simulink model "lab3_ekf_simulation"  (R2023b)
settings: Solver=FixedStepAuto  StartTime=0.0  StopTime=30  RelTol=1e-3
values from neighbouring files (symbols this model uses):
  A_model = A    [lab3_ekf_formulation.m]    (also in lab3_ekf_formulation_vel.m)
  F_linear = A    [lab3_ekf_formulation.m]    (also in lab3_ekf_formulation_vel.m)
  P_init = Q    [lab3_ekf_formulation.m]    (also in lab3_ekf_formulation_vel.m)
  Q = [1 alpha 1/2*alpha ; alpha alpha^2 1/2*alpha^2 ;      1/2*alpha 1/2*alpha^2 1/4*alpha^4]*expected_x_std^2*1e-3    [lab3_ekf_formulation.m]    (also in lab3_ekf_formulation_no_simulink.m = diag([0.2 0.4 1.0])*expected_x_std^2; lab3_ekf_formulation_vel.m = diag([0.2 0.4]))
  R = sensor_noise_var    [lab3_ekf_formulation.m]    (also in lab3_ekf_formulation_no_simulink.m; lab3_ekf_formulation_vel.m)
  sensor_coeffs = coeffs    [lab3_ekf_formulation.m]    (also in lab3_ekf_formulation_no_simulink.m; lab3_ekf_formulation_vel.m)
  T_ekf = 1/nyquist_freq    (= 0.153846153846)    [lab3_ekf_formulation.m]    (also in lab3_ekf_formulation_no_simulink.m = 0.133333333333; lab3_ekf_formulation_vel.m = 1E-4*floor(1/nyquist_freq*1E4))
  x_init = zeros(3,1)    [lab3_ekf_formulation.m]    (also in lab3_ekf_formulation_vel.m = zeros(2,1))
libraries: simulink x2
settings Model: Creator=samuel  LastModifiedBy=samuel

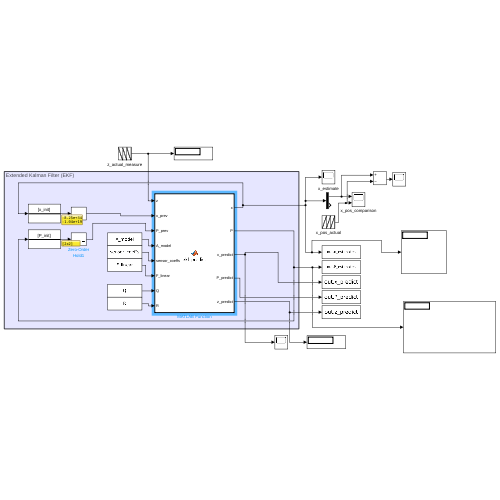
[thumbnail: Simulink's stored preview of the top-level diagram]
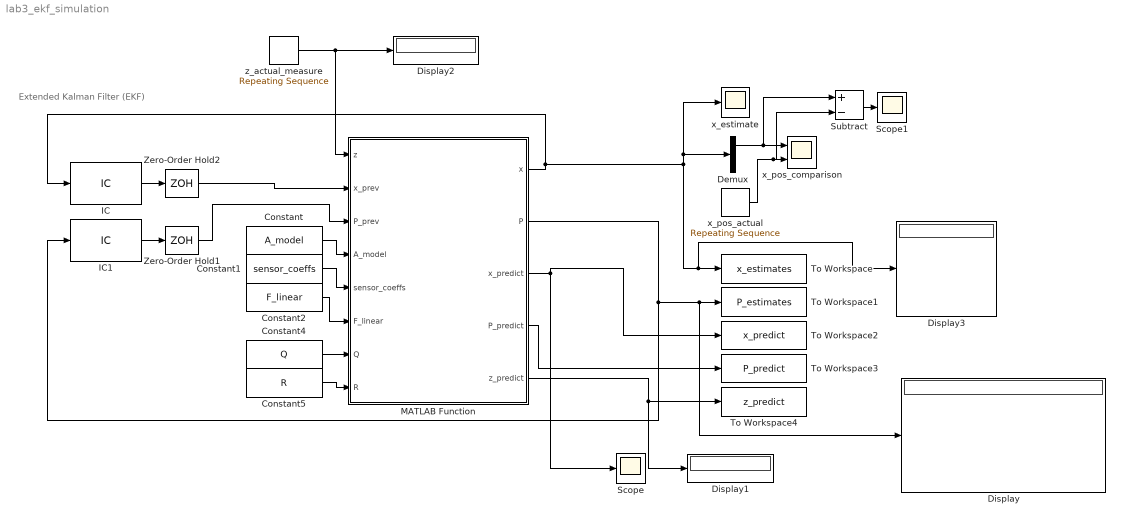
== system lab3_ekf_simulation ==
  note: Extended Kalman Filter (EKF)
  Constant : Constant  Value=A_model  VectorParams1D=off
  Constant1 : Constant  Value=sensor_coeffs
  Constant2 : Constant  Value=F_linear  VectorParams1D=off
  Constant4 : Constant  Value=Q  VectorParams1D=off
  Constant5 : Constant  Value=R  VectorParams1D=off
  Demux : Demux  Outputs=2
  Display{,1..3} (4 alike) : Display
  IC : InitialCondition  Value=x_init
  IC1 : InitialCondition  Value=P_init
  MATLAB Function : MATLAB Function  TreatAsAtomicUnit=on
  Scope : Scope
  Scope1 : Scope
  Subtract : Sum  Inputs=+-
  To Workspace : ToWorkspace  VariableName=x_estimates  SampleTime=-1
  To Workspace1 : ToWorkspace  VariableName=P_estimates  SampleTime=-1
  To Workspace2 : ToWorkspace  VariableName=x_predict  SampleTime=-1
  To Workspace3 : ToWorkspace  VariableName=P_predict  SampleTime=-1
  To Workspace4 : ToWorkspace  VariableName=z_predict  SampleTime=-1
  Zero-Order Hold1 : ZeroOrderHold  SampleTime=T_ekf
  Zero-Order Hold2 : ZeroOrderHold  SampleTime=T_ekf
  x_estimate : Scope
  x_pos_actual : simulink/Sources/Repeating Sequence  rep_seq_t=t_actual  rep_seq_y=x_pos_actual
  x_pos_comparison : Scope  NumInputPorts=2
  z_actual_measure : simulink/Sources/Repeating Sequence  rep_seq_t=t_actual  rep_seq_y=z_actual_measure
  wires:
  MATLAB Function/2(P) -> Display/1, To Workspace1/1, IC1/1
  MATLAB Function/1(x) -> x_estimate/1, Demux/1, Display3/1, To Workspace/1, IC/1
  z_actual_measure/1 -> MATLAB Function/1(z), Display2/1
  Demux/1 -> Subtract/1, x_pos_comparison/1
  x_pos_actual/1 -> Subtract/2, x_pos_comparison/2
  Constant/1 -> MATLAB Function/4(A_model)
  Constant5/1 -> MATLAB Function/8(R)
  Constant4/1 -> MATLAB Function/7(Q)
  Constant2/1 -> MATLAB Function/6(F_linear)
  Constant1/1 -> MATLAB Function/5(sensor_coeffs)
  IC/1 -> Zero-Order Hold2/1
  IC1/1 -> Zero-Order Hold1/1
  Zero-Order Hold1/1 -> MATLAB Function/3(P_prev)
  Zero-Order Hold2/1 -> MATLAB Function/2(x_prev)
  MATLAB Function/3(x_predict) -> To Workspace2/1, Scope/1
  MATLAB Function/4(P_predict) -> To Workspace3/1
  MATLAB Function/5(z_predict) -> Display1/1, To Workspace4/1
  Subtract/1 -> Scope1/1

== matlab function lab3_ekf_simulation/MATLAB Function ==
  data: z input; x_prev input; P_prev input; x output; P output; A_model input; sensor_coeffs input; F_linear input; Q input; R input; x_predict output; P_predict output; z_predict output
function [x,P,x_predict,P_predict,z_predict] = ekf_predict(z,x_prev,P_prev,...
    A_model,sensor_coeffs,F_linear,Q,R)

x = zeros(size(x_prev));
P = zeros(size(P_prev));

% sensor coefficients
a = sensor_coeffs(1);
b = sensor_coeffs(2);
c = sensor_coeffs(3);
d = sensor_coeffs(4);

% predict states (x in cm, note sensor model accepts mm)
x_predict = A_model*x_prev;
z_predict = (a*x_prev(1)+b)/(c*x_prev(1)+d);

% predict estimation covariance
P_predict = F_linear*P_prev*F_linear' + Q;

% kalman gain
H_linear = [((-b*c+a*d)/(c*x_predict(1)+d)^2) 0]
K = P_predict*H_linear'*(H_linear*P_predict*H_linear' + R)^-1;

% update state estimation
x = x_predict + K*(z - z_predict);
P = (eye(size(P))-K*H_linear)*P_predict;
